simulink model "mux"  (Simulink 7.3)
settings: Solver=FixedStepDiscrete  StartTime=0.0  StopTime=10.0  FixedStep=1  RelTol=1e-3
settings Model: Creator=ksmyth  LastModifiedBy=hnine
settings OptimizationCC: InitFltsAndDblsToZero=on
settings DebuggingCC: SaveWithParameterizedLinksMsg=none
settings GRTTargetCC: TargetFcnLib=ansi_tfl_tmw.mat

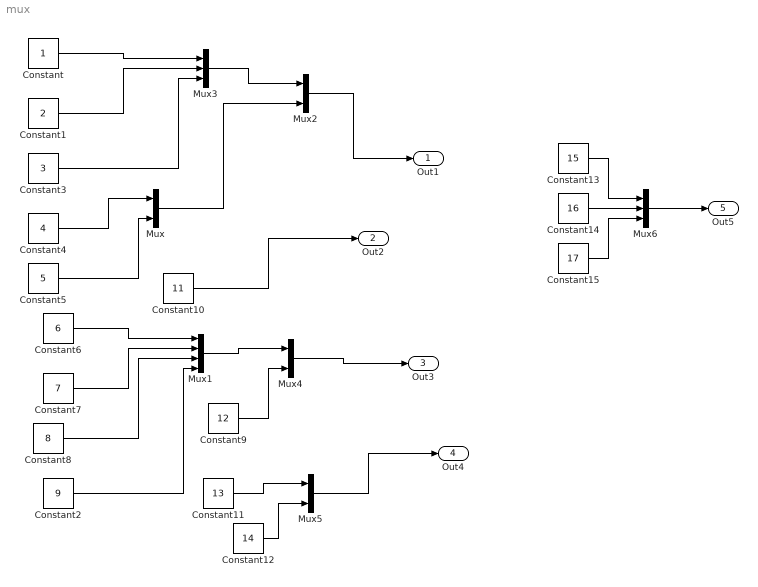
== system mux ==
  Constant : Constant  OutDataType=sfix(16)  OutScaling=2^0
  Constant1 : Constant  Value=2  OutDataType=sfix(16)  OutScaling=2^0
  Constant10 : Constant  Value=11  OutDataType=sfix(16)  OutScaling=2^0
  Constant11 : Constant  Value=13  OutDataType=sfix(16)  OutScaling=2^0
  Constant12 : Constant  Value=14  OutDataType=sfix(16)  OutScaling=2^0
  Constant13 : Constant  Value=15  OutDataType=sfix(16)  OutScaling=2^0
  Constant14 : Constant  Value=16  OutDataType=sfix(16)  OutScaling=2^0
  Constant15 : Constant  Value=17  OutDataType=sfix(16)  OutScaling=2^0
  Constant2 : Constant  Value=9  OutDataType=sfix(16)  OutScaling=2^0
  Constant3 : Constant  Value=3  OutDataType=sfix(16)  OutScaling=2^0
  Constant4 : Constant  Value=4  OutDataType=sfix(16)  OutScaling=2^0
  Constant5 : Constant  Value=5  OutDataType=sfix(16)  OutScaling=2^0
  Constant6 : Constant  Value=6  OutDataType=sfix(16)  OutScaling=2^0
  Constant7 : Constant  Value=7  OutDataType=sfix(16)  OutScaling=2^0
  Constant8 : Constant  Value=8  OutDataType=sfix(16)  OutScaling=2^0
  Constant9 : Constant  Value=12  OutDataType=sfix(16)  OutScaling=2^0
  Mux{,2,4..5} (4 alike) : Mux  Inputs=2
  Mux1 : Mux
  Mux3 : Mux  Inputs=3
  Mux6 : Mux  Inputs=3
  Out1 : Outport  OutDataType=sfix(16)  OutScaling=2^0
  Out2 : Outport  Port=2  OutDataType=sfix(16)  OutScaling=2^0
  Out3 : Outport  Port=3  OutDataType=sfix(16)  OutScaling=2^0
  Out4 : Outport  Port=4  OutDataType=sfix(16)  OutScaling=2^0
  Out5 : Outport  Port=5  PortDimensions=3  DataType=double  OutDataType=sfix(16)  OutScaling=2^0  OutDataTypeStr=double
  wires:
  Constant/1 -> Mux3/1
  Constant1/1 -> Mux3/2
  Constant3/1 -> Mux3/3
  Constant4/1 -> Mux/1
  Constant5/1 -> Mux/2
  Mux3/1 -> Mux2/1
  Mux/1 -> Mux2/2
  Mux2/1 -> Out1/1
  Constant6/1 -> Mux1/1
  Constant7/1 -> Mux1/2
  Constant8/1 -> Mux1/3
  Constant2/1 -> Mux1/4
  Mux1/1 -> Mux4/1
  Constant9/1 -> Mux4/2
  Mux4/1 -> Out3/1
  Constant10/1 -> Out2/1
  Constant11/1 -> Mux5/1
  Mux5/1 -> Out4/1
  Constant12/1 -> Mux5/2
  Constant13/1 -> Mux6/1
  Constant14/1 -> Mux6/2
  Constant15/1 -> Mux6/3
  Mux6/1 -> Out5/1
